simulink model "Loops7"  (Simulink 6.0)
settings: Solver=ode45  StartTime=0.0  StopTime=10.0  RelTol=1e-3
settings Model: Creator=scaife  LastModifiedBy=scaife  ExtModeAutoUpdateStatusClock=off
settings DataIOCC: SignalLoggingName=sigsOut
settings DebuggingCC: SolverPrmCheckMsg=none
settings HardwareCC: TargetUnknown=on
settings STFCustomTargetCC: TargetFcnLib=ansi_tfl_tmw.mat  GenFloatMathFcnCalls=ANSI_C  ModelReferenceCompliant=off  SystemTargetFile=grt.tlc

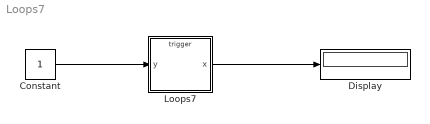
== system Loops7 ==
  Constant : Constant
  Display : Display
  Loops7 : Stateflow chart
  wires:
  Loops7/1(x) -> Display/1
  Constant/1 -> Loops7/1(y)

== stateflow chart Loops7 ==
  state A
  state B
  A -> (junction 5) : {x=0}
  (junction 6) -> B
  (default) -> A
  (junction 5) -> (junction 7)
  (junction 7) -> (junction 6) : {x++}
  (junction 5) -> (junction 5) : [x<3]{x++}
  (junction 6) -> (junction 7) : [x<6]
  data: x output int32; y input double
  events: event input EITHER_EDGE_EVENT
